simulink library "AEBSStateMachineLib"  (R2020b)
settings: Solver=VariableStepAuto  StartTime=0.0  StopTime=10.0  RelTol=1e-3
undefined symbols (not defined in the file): ModSts
libraries: simulink x2
settings Model: Creator=Acer  LastModifiedBy=Acer
settings DataIOCC: ReturnWorkspaceOutputs=off
settings DebuggingCC: ArithmeticOperatorsInVariantConditions=warning
settings SFSimCC: SimUseLocalCustomCode=off  CustomCodeUndefinedFunction=UseInterfaceOnly
settings RTWCC: RTWUseLocalCustomCode=off
settings CodeAppCC: StateflowObjectComments=on

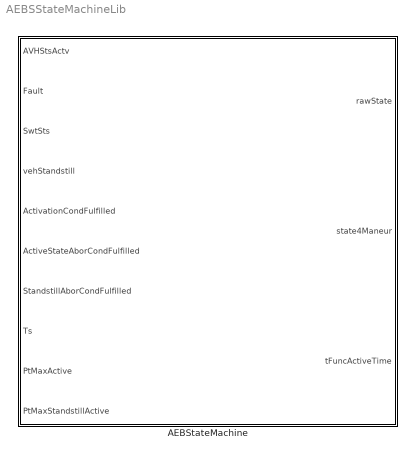
== system AEBSStateMachineLib ==
  AEBStateMachine : Subsystem

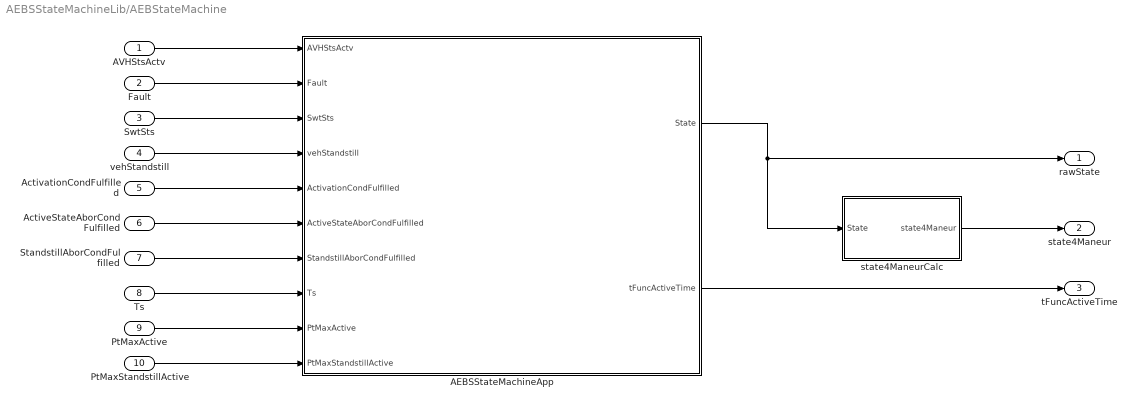
== system AEBSStateMachineLib/AEBStateMachine ==
  AVHStsActv : Inport
  Fault : Inport  Port=2
  SwtSts : Inport  Port=3
  vehStandstill : Inport  Port=4
  ActivationCondFulfilled : Inport  Port=5
  ActiveStateAborCondFulfilled : Inport  Port=6
  StandstillAborCondFulfilled : Inport  Port=7
  Ts : Inport  Port=8
  PtMaxActive : Inport  Port=9
  PtMaxStandstillActive : Inport  Port=10
  AEBSStateMachineApp : Stateflow chart  TreatAsAtomicUnit=on
  state4ManeurCalc : Subsystem
  rawState : Outport
  state4Maneur : Outport  Port=2
  tFuncActiveTime : Outport  Port=3
  wires:
  ActivationCondFulfilled/1 -> AEBSStateMachineApp/5(ActivationCondFulfilled)
  ActiveStateAborCondFulfilled/1 -> AEBSStateMachineApp/6(ActiveStateAborCondFulfilled)
  StandstillAborCondFulfilled/1 -> AEBSStateMachineApp/7(StandstillAborCondFulfilled)
  Ts/1 -> AEBSStateMachineApp/8(Ts)
  PtMaxStandstillActive/1 -> AEBSStateMachineApp/10(PtMaxStandstillActive)
  PtMaxActive/1 -> AEBSStateMachineApp/9(PtMaxActive)
  AEBSStateMachineApp/1(State) -> state4ManeurCalc/1(State), rawState/1
  AEBSStateMachineApp/2(tFuncActiveTime) -> tFuncActiveTime/1
  state4ManeurCalc/1(state4Maneur) -> state4Maneur/1
  AVHStsActv/1 -> AEBSStateMachineApp/1(AVHStsActv)
  Fault/1 -> AEBSStateMachineApp/2(Fault)
  SwtSts/1 -> AEBSStateMachineApp/3(SwtSts)
  vehStandstill/1 -> AEBSStateMachineApp/4(vehStandstill)

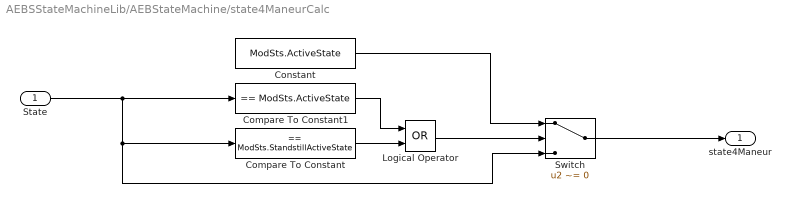
== system AEBSStateMachineLib/AEBStateMachine/state4ManeurCalc ==
  State : Inport
  Compare To Constant : simulink/Logic and Bit Operations/Compare To Constant  relop===  const=ModSts.StandstillActiveState  OutDataTypeStr=boolean
  Compare To Constant1 : simulink/Logic and Bit Operations/Compare To Constant  relop===  const=ModSts.ActiveState  OutDataTypeStr=boolean
  Constant : Constant  Value=ModSts.ActiveState  OutDataTypeStr=Enum: ModSts
  Logical Operator : Logic  Operator=OR  AllPortsSameDT=off  OutDataTypeStr=boolean
  Switch : Switch  Criteria=u2 ~= 0
  state4Maneur : Outport
  wires:
  Constant/1 -> Switch/1
  Switch/1 -> state4Maneur/1
  State/1 -> Compare To Constant/1, Switch/3, Compare To Constant1/1
  Compare To Constant/1 -> Logical Operator/2
  Compare To Constant1/1 -> Logical Operator/1
  Logical Operator/1 -> Switch/2

== stateflow chart AEBSStateMachineLib/AEBStateMachine/AEBSStateMachineApp ==
  state PassiveState
    state OFFState
      en,du:
      State = ModSts.OFFState;
    state StandbyState
      en,du:
      State = ModSts.StandbyState;
    (default) -> (junction 17)
    (junction 17) -> OFFState [order 1] : [SwtSts == OFF]
    (junction 17) -> StandbyState [order 2]
    OFFState -> StandbyState : [SwtSts == ON]
    StandbyState -> OFFState [order 2] : [SwtSts == OFF]
  state FaultState
    en,du:
    State = ModSts.FaultState;
  state ActiveMainState
    en:
    %State = ModSts.ActiveState;
    tFuncActiveTime = 0;
    du:
    %State = ModSts.ActiveState;
    tFuncActiveTime += Ts;
    exit:
    tFuncActiveTime = 0;
    state ActiveControlState
      en:
      State = ModSts.ActiveState;
      tActiveState = 0;
      du:
      State = ModSts.ActiveState;
      tActiveState += Ts;
      exit:
      tActiveState = 0;
    state StandstillActiveState
      en:
      State = ModSts.StandstillActiveState;
      tStandstillState = 0;
      du:
      State = ModSts.StandstillActiveState;
      tStandstillState += Ts;
      exit:
      tStandstillState = 0;
    (junction 32) -> (junction 35)
    (junction 33) -> (junction 35)
    ActiveControlState -> (junction 32) [order 1] : [	SwtSts == OFF || ...
        | 	ActiveStateAborCondFulfilled == true || ...
        | 	tActiveState > PtMaxActive
        | ]
    StandstillActiveState -> (junction 33) : [
        | 	SwtSts == OFF || ...
        |       AVHStsActv ==  true||...
        | 	StandstillAborCondFulfilled == true ||...
        | 	tStandstillState > PtMaxStandstillActive
        | ]
    (default) -> ActiveControlState
    ActiveControlState -> StandstillActiveState [order 2] : [vehStandstill == true]
  (default) -> PassiveState
  FaultState -> PassiveState : [Fault == false]
  PassiveState -> FaultState : [Fault == true]
  StandbyState -> ActiveMainState [order 1] : [ActivationCondFulfilled == true]
  (junction 23) -> FaultState
  (junction 35) -> PassiveState
  ActiveMainState -> (junction 23) : [Fault == true]
  data: AVHStsActv input boolean; Fault input; SwtSts input; vehStandstill input; ActivationCondFulfilled input; ActiveStateAborCondFulfilled input; StandstillAborCondFulfilled input; Ts input; PtMaxActive input; PtMaxStandstillActive input; State output Enum: ModSts; OFF parameter; ON parameter; tActiveState local double; tStandstillState local double; tFuncActiveTime output double
